simulink model "Lab5_StartModel_20192020"  (R2013a)
settings: Solver=ode45  SolverMode=SingleTasking  StartTime=0.0  StopTime=1  MaxStep=0.01  RelTol=1e-2
libraries: fl_lib x13, nesl_utility x7, elec_lib x1
settings Model: Creator=Nic  LastModifiedBy=ncleju
settings DataIOCC: SignalLoggingSaveFormat=ModelDataLogs
settings OptimizationCC: BlockReduction=off  BooleanDataType=off
settings DebuggingCC: SaveWithParameterizedLinksMsg=none  SignalResolutionControl=TryResolveAllWithWarning  SolverPrmCheckMsg=none  MultiTaskDSMMsg=warning  MultiTaskCondExecSysMsg=none  FrameProcessingCompatibilityMsg=error
settings HardwareCC: TargetUnknown=on
settings GRTTargetCC: CodeReplacementLibrary=C89/C90 (ANSI)
settings SimscapeCC: SimscapeNormalizeSystem=off
settings ConfigurationSet: Description=Simscape Multibody

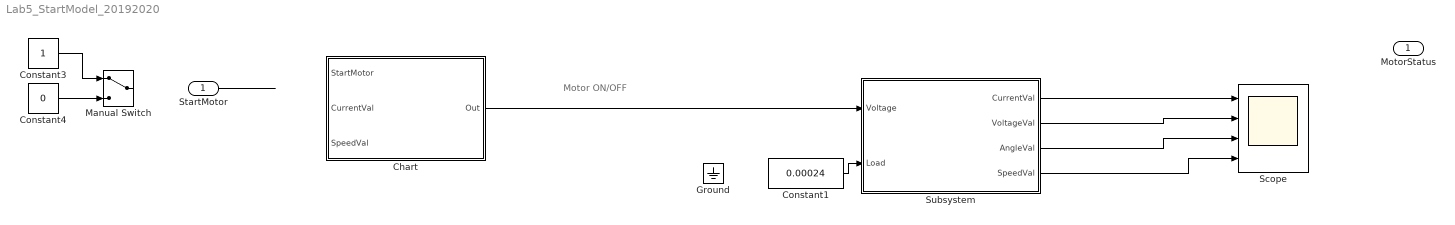
== system Lab5_StartModel_20192020 ==
  note: Motor ON/OFF
  StartMotor : Inport
  Chart : Stateflow chart  TreatAsAtomicUnit=on
      settings: PermitHierarchicalResolution=ParametersOnly
  Constant1 : Constant  Value=0.00024
  Constant3 : Constant
  Constant4 : Constant  Value=0
  Ground : Ground
  Manual Switch : ManualSwitch
  Scope : Scope  NumInputPorts=4
      settings: TimeRange=auto  LimitDataPoints=on  MaxDataPoints=5000  SaveToWorkspace=off  SaveName=ScopeData  YMin=-1~0~-25~-750  YMax=18~11~425~750  SampleTime=-1  DataFormat=Array
  Subsystem : Subsystem
  MotorStatus : Outport
  wires:
  Subsystem/1(CurrentVal) -> Scope/1
  Subsystem/2(VoltageVal) -> Scope/2
  Subsystem/3("AngleVal\t") -> Scope/3
  Subsystem/4(SpeedVal) -> Scope/4
  Constant1/1 -> Subsystem/2(Load)
  Chart/1(Out) -> Subsystem/1(Voltage)
  StartMotor/1 -> ?
  ? -> MotorStatus/1
  Constant4/1 -> Manual Switch/2
  Constant3/1 -> Manual Switch/1

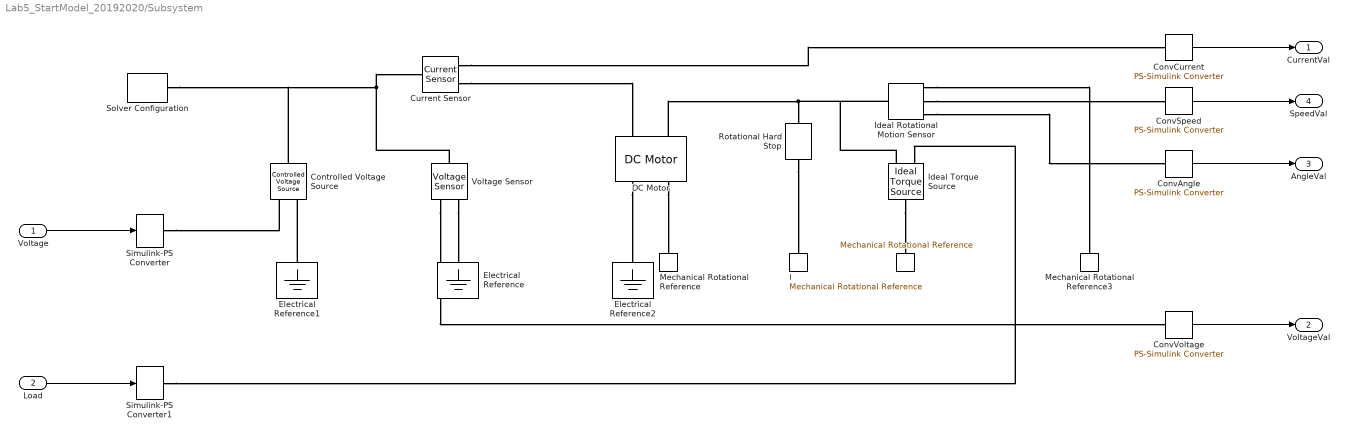
== system Lab5_StartModel_20192020/Subsystem ==
  Voltage : Inport
  Load : Inport  Port=2
  " " : fl_lib/Mechanical/Rotational Elements/Mechanical Rotational Reference
  Controlled Voltage Source : fl_lib/Electrical/Electrical Sources/Controlled Voltage Source
  ConvAngle : nesl_utility/PS-Simulink Converter  PhysicalDomain=network_engine_domain  SubClassName=ps_output  LeftPortType=input  RightPortType=output  PseudoPeriodic=off  Frequencies=[]  AffineConversion=off
  ConvCurrent : nesl_utility/PS-Simulink Converter  PhysicalDomain=network_engine_domain  SubClassName=ps_output  LeftPortType=input  RightPortType=output  PseudoPeriodic=off  Frequencies=[]  AffineConversion=off
  ConvSpeed : nesl_utility/PS-Simulink Converter  PhysicalDomain=network_engine_domain  SubClassName=ps_output  LeftPortType=input  RightPortType=output  PseudoPeriodic=off  Frequencies=[]  AffineConversion=off
  ConvVoltage : nesl_utility/PS-Simulink Converter  PhysicalDomain=network_engine_domain  SubClassName=ps_output  LeftPortType=input  RightPortType=output  PseudoPeriodic=off  Frequencies=[]  AffineConversion=off
  Current Sensor : fl_lib/Electrical/Electrical Sensors/Current Sensor
  DC Motor : elec_lib/Actuators & Drivers/Rotational Actuators/DC Motor  parameterization=1  Ra=0.83 Ohm  La=0.63 mH  emf_or_torque=1  Kv=0.00191 V/rpm  Ki=6.876e-4 N*m/A  T_stall=2.4e-4 N*m  w_max=1.91e+4 rpm  w_rated=1.5e+4 rpm  P_rated=0.08 W  V_rated=1.5 V  J=4.2E-06 kg*m^2  lam_param=1  lam=0 N*m/(rad/s)  i_noload=0 A  V_i_noload=1.5 V  speed0=0 rpm  alpha=0.00393 1/K  Tmeas=25 C  thermal_mass=100 J/K  initial_temperature=25 C
  Electrical Reference : fl_lib/Electrical/Electrical Elements/Electrical Reference
  Electrical Reference1 : fl_lib/Electrical/Electrical Elements/Electrical Reference
  Electrical Reference2 : fl_lib/Electrical/Electrical Elements/Electrical Reference
  Ideal Rotational Motion Sensor : fl_lib/Mechanical/Mechanical Sensors/Ideal Rotational Motion Sensor  offset=0 rad
  Ideal Torque Source : fl_lib/Mechanical/Mechanical Sources/Ideal Torque Source
  Mechanical Rotational Reference : fl_lib/Mechanical/Rotational Elements/Mechanical Rotational Reference
  Mechanical Rotational Reference3 : fl_lib/Mechanical/Rotational Elements/Mechanical Rotational Reference
  Rotational Hard Stop : fl_lib/Mechanical/Rotational Elements/Rotational Hard Stop  upper_bnd=400 rad  lower_bnd=-400 rad  stiff_up=1e6 N*m/rad  stiff_low=1e6 N*m/rad  D_up=0.01 N*m/(rad/s)  D_low=0.01 N*m/(rad/s)  model=3  transition=0.001 rad  w_specify=off  w_priority=None  w=0 rad/s  w_nominal_specify=off  w_nominal_unit=rad/s  w_nominal_value=1  t_specify=off  t_priority=None  t=0 N*m  t_nominal_specify=off  t_nominal_unit=N*m  t_nominal_value=1  phi_specify=on  phi_priority=High  phi=0 rad  phi_nominal_specify=off  phi_nominal_unit=rad  phi_nominal_value=1
  Simulink-PS Converter : nesl_utility/Simulink-PS Converter  PhysicalDomain=network_engine_domain  SubClassName=ps_input  LeftPortType=input  RightPortType=output  PseudoPeriodic=off  Frequencies=[]  NoiseDistribution=none  NoiseParameters=[]  AffineConversion=off  FilteringAndDerivatives=zero  SimscapeFilterOrder=1  InputFilterTimeConstant=0.001  UdotUserProvided=1
  Simulink-PS Converter1 : nesl_utility/Simulink-PS Converter  PhysicalDomain=network_engine_domain  SubClassName=ps_input  LeftPortType=input  RightPortType=output  PseudoPeriodic=off  Frequencies=[]  NoiseDistribution=none  NoiseParameters=[]  AffineConversion=off  FilteringAndDerivatives=zero  SimscapeFilterOrder=1  InputFilterTimeConstant=0.001  UdotUserProvided=1
  Solver Configuration : nesl_utility/Solver Configuration  PhysicalDomain=network_engine_domain  SubClassName=solver  LeftPortType=input  RightPortType=generic  Tones=[]  Harmonics=[]  SimulateNoise=off  Profile=off  UseLocalSampling=off  EnableSwitchedLinearOptims=on  FrequencyDomain=off  UseCCode=off  RelTol=0.001  AbsTol=1e-06  MinStep=1e-09  ToWorkspace=off  RevertToSquareIcSolve=off  NumHomotopyIterations=100  PhasorMode=off  PhasorModeNumHarmonics=1  DoDC=off  ResidualTolerance=1e-09  UseLocalSolver=off  LocalSolverChoice=NE_BACKWARD_EULER_ADVANCER  LocalSolverSampleTime=0.001  DoFixedCost=off  MaxNonlinIter=3  MaxModeIter=2  LinearAlgebra=Sparse  EquationFormulation=NE_TIME_EF  DelaysMemoryBudget=1024  AutomaticFiltering=on  FilteringTimeConstant=0.001  PartitionStorageMethod=AS_NEEDED  PartitionMemoryBudget=1024
  Voltage Sensor : fl_lib/Electrical/Electrical Sensors/Voltage Sensor
  "l " : fl_lib/Mechanical/Rotational Elements/Mechanical Rotational Reference
  CurrentVal : Outport
  VoltageVal : Outport  Port=2
  "AngleVal\t" : Outport  Port=3
  SpeedVal : Outport  Port=4
  wires:
  ConvVoltage/1 -> VoltageVal/1
  Voltage/1 -> Simulink-PS Converter/1
  Load/1 -> Simulink-PS Converter1/1
  ConvCurrent/1 -> CurrentVal/1
  ConvAngle/1 -> "AngleVal\t"/1
  ConvSpeed/1 -> SpeedVal/1
  connections:
  Voltage Sensor/RConn1 -- ConvVoltage/LConn1
  Voltage Sensor/RConn2 -- Electrical Reference/LConn1
  Voltage Sensor/LConn1 -- Controlled Voltage Source/LConn1 -- Solver Configuration/RConn1 -- Current Sensor/LConn1
  DC Motor/RConn2 -- Mechanical Rotational Reference/LConn1
  Simulink-PS Converter/RConn1 -- Controlled Voltage Source/RConn1
  Simulink-PS Converter1/RConn1 -- Ideal Torque Source/RConn1
  Ideal Rotational Motion Sensor/RConn1 -- Mechanical Rotational Reference3/LConn1
  DC Motor/RConn1 -- Electrical Reference2/LConn1
  Current Sensor/RConn1 -- ConvCurrent/LConn1
  Current Sensor/RConn2 -- DC Motor/LConn1
  Rotational Hard Stop/RConn1 -- "l "/LConn1
  Ideal Torque Source/LConn1 -- " "/LConn1
  DC Motor/LConn2 -- Ideal Torque Source/RConn2 -- Ideal Rotational Motion Sensor/LConn1 -- Rotational Hard Stop/LConn1
  Ideal Rotational Motion Sensor/RConn3 -- ConvAngle/LConn1
  Ideal Rotational Motion Sensor/RConn2 -- ConvSpeed/LConn1
  Electrical Reference1/LConn1 -- Controlled Voltage Source/RConn2

== stateflow chart Lab5_StartModel_20192020/Chart ==
  data: StartMotor input; CurrentVal input; SpeedVal input; Out output double
